simulink model "Fb_lin_control_hovering"  (R2021b)
settings: Solver=ode4  StartTime=0.0  StopTime=10.0  FixedStep=1e-4  RelTol=1e-3
settings Model: Creator=pierg  LastModifiedBy=pierg
settings ModelReferenceCC: ModelReferenceMinAlgLoopOccurrences=on

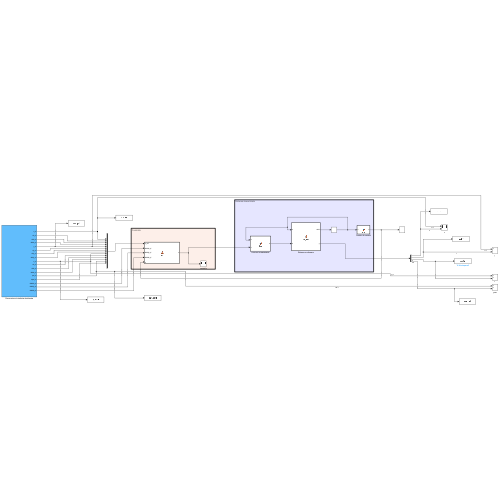
[thumbnail: Simulink's stored preview of the top-level diagram]
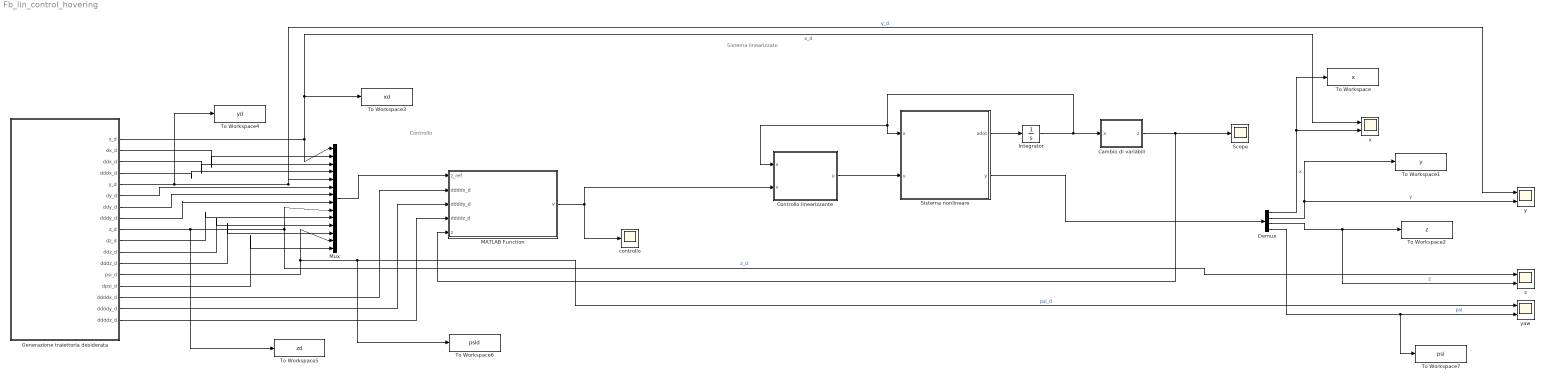
== system Fb_lin_control_hovering ==
  note: Controllo
  note: Sistema linearizzato
  Cambio di variabili : MATLAB Function  TreatAsAtomicUnit=on
  Controllo linearizzante : MATLAB Function  TreatAsAtomicUnit=on
  Demux : Demux
  Generazione traiettoria desiderata : Subsystem
  Integrator : Integrator  InitialCondition=[10 5 5 0 0 0 0 0 pi/4 0 0 0 9.81*2 0]'
  MATLAB Function : MATLAB Function  TreatAsAtomicUnit=on
  Mux : Mux  Inputs=14
  Scope : Scope
  Sistema nonlineare : MATLAB Function  TreatAsAtomicUnit=on
  To Workspace : ToWorkspace  VariableName=x  SaveFormat=Structure  SampleTime=-1
  To Workspace1 : ToWorkspace  VariableName=y  SaveFormat=Structure  SampleTime=-1
  To Workspace2 : ToWorkspace  VariableName=z  SaveFormat=Structure  SampleTime=-1
  To Workspace3 : ToWorkspace  VariableName=xd  SaveFormat=Structure  SampleTime=-1
  To Workspace4 : ToWorkspace  VariableName=yd  SaveFormat=Structure  SampleTime=-1
  To Workspace5 : ToWorkspace  VariableName=zd  SaveFormat=Structure  SampleTime=-1
  To Workspace6 : ToWorkspace  VariableName=psid  SaveFormat=Structure  SampleTime=-1
  To Workspace7 : ToWorkspace  VariableName=psi  SaveFormat=Structure  SampleTime=-1
  controllo : Scope
  x : Scope  NumInputPorts=2
  y : Scope  NumInputPorts=2
  yaw : Scope  NumInputPorts=2
  z : Scope  NumInputPorts=2
  wires:
  Sistema nonlineare/1(xdot) -> Integrator/1
  Integrator/1 -> Cambio di variabili/1(x), Controllo linearizzante/1(x), Sistema nonlineare/1(x)
  Controllo linearizzante/1(u) -> Sistema nonlineare/2(u)
  Sistema nonlineare/2(y) -> Demux/1
  Demux/1 -> To Workspace/1, x/2  "x"
  Demux/2 -> To Workspace1/1, y/2  "y"
  Demux/3 -> To Workspace2/1, z/2  "z"
  Cambio di variabili/1(z) -> MATLAB Function/5(z), Scope/1
  MATLAB Function/1(v) -> controllo/1, Controllo linearizzante/2(v)
  Generazione traiettoria desiderata/9(z_d) -> To Workspace5/1, Mux/9, z/1  "z_d"
  Generazione traiettoria desiderata/8(dddy_d) -> Mux/8
  Generazione traiettoria desiderata/10(dz_d) -> Mux/10
  Generazione traiettoria desiderata/7(ddy_d) -> Mux/7
  Generazione traiettoria desiderata/11(ddz_d) -> Mux/11
  Generazione traiettoria desiderata/6(dy_d) -> Mux/6
  Generazione traiettoria desiderata/12(dddz_d) -> Mux/12
  Generazione traiettoria desiderata/5(y_d) -> To Workspace4/1, y/1, Mux/5  "y_d"
  Generazione traiettoria desiderata/13(psi_d) -> To Workspace6/1, yaw/1, Mux/13  "psi_d"
  Generazione traiettoria desiderata/4(dddx_d) -> Mux/4
  Generazione traiettoria desiderata/14(dpsi_d) -> Mux/14
  Generazione traiettoria desiderata/3(ddx_d) -> Mux/3
  Generazione traiettoria desiderata/2(dx_d) -> Mux/2
  Generazione traiettoria desiderata/1(x_d) -> To Workspace3/1, x/1, Mux/1  "x_d"
  Mux/1 -> MATLAB Function/1(z_ref)
  Generazione traiettoria desiderata/15(ddddx_d) -> MATLAB Function/2(ddddx_d)
  Generazione traiettoria desiderata/16(ddddy_d) -> MATLAB Function/3(ddddy_d)
  Generazione traiettoria desiderata/17(ddddz_d) -> MATLAB Function/4(ddddz_d)
  Demux/4 -> To Workspace7/1, yaw/2  "psi"

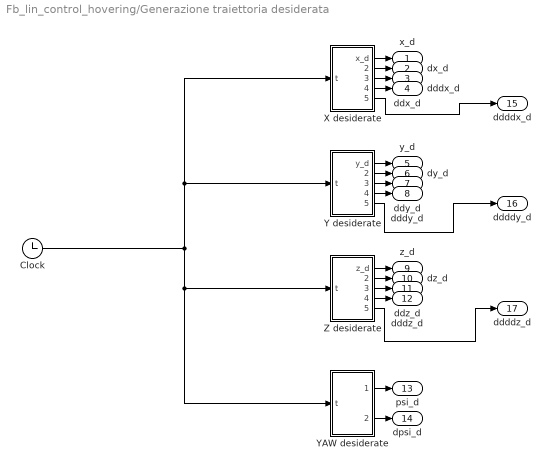
== system Fb_lin_control_hovering/Generazione traiettoria desiderata ==
  Clock : Clock
  X desiderate : Subsystem
  Y desiderate : Subsystem
  YAW desiderate : Subsystem
  Z desiderate : Subsystem
  x_d : Outport
  dx_d : Outport  Port=2
  ddx_d : Outport  Port=3
  dddx_d : Outport  Port=4
  y_d : Outport  Port=5
  dy_d : Outport  Port=6
  ddy_d : Outport  Port=7
  dddy_d : Outport  Port=8
  z_d : Outport  Port=9
  dz_d : Outport  Port=10
  ddz_d : Outport  Port=11
  dddz_d : Outport  Port=12
  psi_d : Outport  Port=13
  dpsi_d : Outport  Port=14
  ddddx_d : Outport  Port=15
  ddddy_d : Outport  Port=16
  ddddz_d : Outport  Port=17
  wires:
  Y desiderate/1(y_d) -> y_d/1
  Y desiderate/2(dy_d) -> dy_d/1
  X desiderate/5(ddddx_d) -> ddddx_d/1
  X desiderate/3(ddx_d) -> ddx_d/1
  YAW desiderate/2(dpsi_d) -> dpsi_d/1
  Z desiderate/1(z_d) -> z_d/1
  Z desiderate/4(dddz_d) -> dddz_d/1
  X desiderate/2(dx_d) -> dx_d/1
  Y desiderate/4(dddy_d) -> dddy_d/1
  X desiderate/4(dddx_d) -> dddx_d/1
  Y desiderate/3(ddy_d) -> ddy_d/1
  X desiderate/1(x_d) -> x_d/1
  Z desiderate/5(ddddz_d) -> ddddz_d/1
  Z desiderate/2(dz_d) -> dz_d/1
  YAW desiderate/1(psi_d) -> psi_d/1
  Z desiderate/3(ddz_d) -> ddz_d/1
  Y desiderate/5(ddddy_d) -> ddddy_d/1
  Clock/1 -> YAW desiderate/1(t), Z desiderate/1(t), X desiderate/1(t), Y desiderate/1(t)

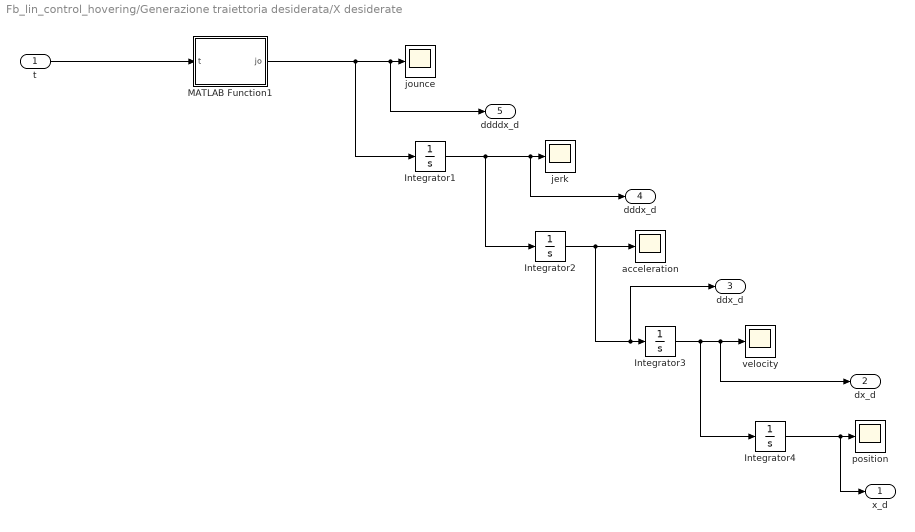
== system Fb_lin_control_hovering/Generazione traiettoria desiderata/X desiderate ==
  t : Inport
  Integrator1 : Integrator
  Integrator2 : Integrator
  Integrator3 : Integrator
  Integrator4 : Integrator  InitialCondition=10
  MATLAB Function1 : MATLAB Function  TreatAsAtomicUnit=on
  acceleration : Scope
  jerk : Scope
  jounce : Scope
  position : Scope
  velocity : Scope
  x_d : Outport
  dx_d : Outport  Port=2
  ddx_d : Outport  Port=3
  dddx_d : Outport  Port=4
  ddddx_d : Outport  Port=5
  wires:
  MATLAB Function1/1(jo) -> Integrator1/1, ddddx_d/1, jounce/1
  Integrator4/1 -> x_d/1, position/1
  Integrator3/1 -> Integrator4/1, dx_d/1, velocity/1
  Integrator2/1 -> ddx_d/1, Integrator3/1, acceleration/1
  Integrator1/1 -> Integrator2/1, dddx_d/1, jerk/1
  t/1 -> MATLAB Function1/1(t)

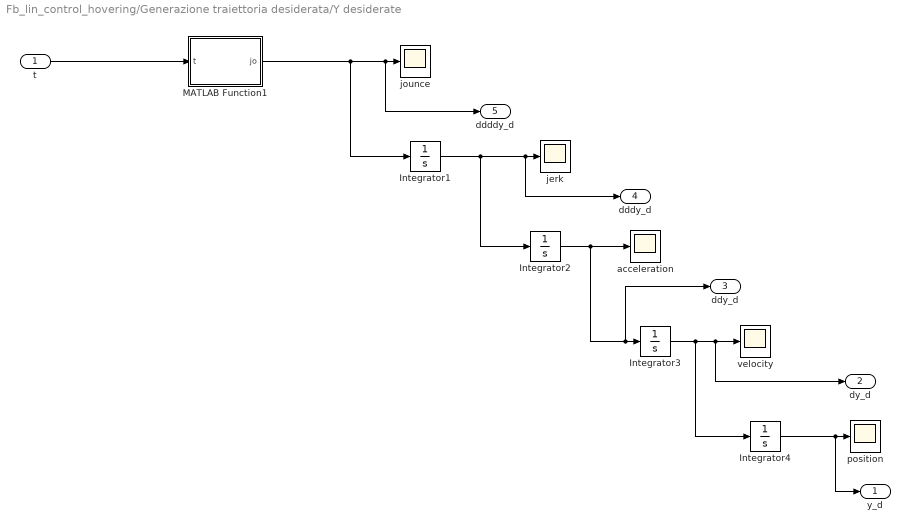
== system Fb_lin_control_hovering/Generazione traiettoria desiderata/Y desiderate ==
  t : Inport
  Integrator1 : Integrator
  Integrator2 : Integrator
  Integrator3 : Integrator
  Integrator4 : Integrator  InitialCondition=5
  MATLAB Function1 : MATLAB Function  TreatAsAtomicUnit=on
  acceleration : Scope
  jerk : Scope
  jounce : Scope
  position : Scope
  velocity : Scope
  y_d : Outport
  dy_d : Outport  Port=2
  ddy_d : Outport  Port=3
  dddy_d : Outport  Port=4
  ddddy_d : Outport  Port=5
  wires:
  t/1 -> MATLAB Function1/1(t)
  Integrator1/1 -> jerk/1, dddy_d/1, Integrator2/1
  Integrator2/1 -> acceleration/1, Integrator3/1, ddy_d/1
  Integrator3/1 -> velocity/1, dy_d/1, Integrator4/1
  Integrator4/1 -> position/1, y_d/1
  MATLAB Function1/1(jo) -> jounce/1, ddddy_d/1, Integrator1/1

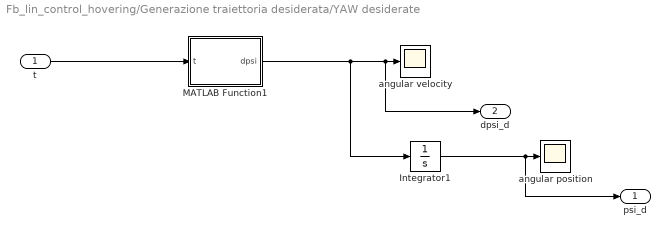
== system Fb_lin_control_hovering/Generazione traiettoria desiderata/YAW desiderate ==
  t : Inport
  Integrator1 : Integrator
  MATLAB Function1 : MATLAB Function  TreatAsAtomicUnit=on
  angular position : Scope
  angular velocity : Scope
  psi_d : Outport
  dpsi_d : Outport  Port=2
  wires:
  t/1 -> MATLAB Function1/1(t)
  Integrator1/1 -> angular position/1, psi_d/1
  MATLAB Function1/1(dpsi) -> angular velocity/1, dpsi_d/1, Integrator1/1

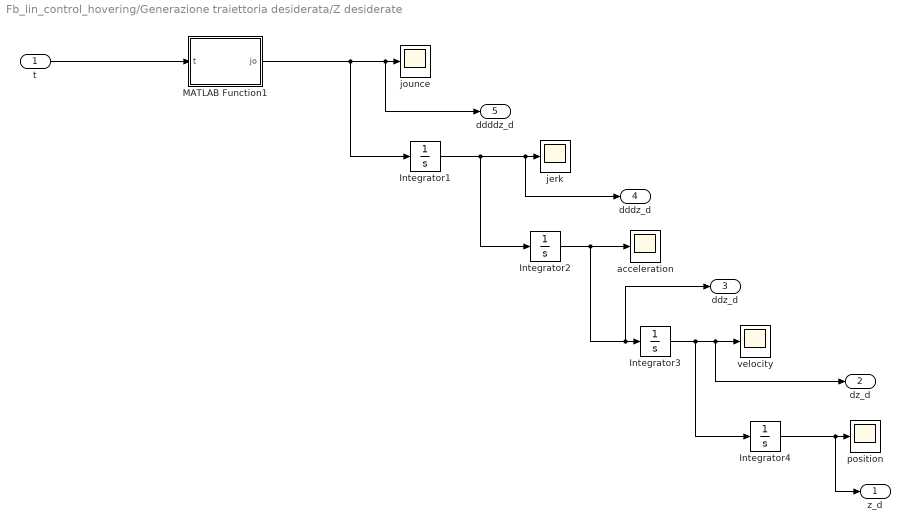
== system Fb_lin_control_hovering/Generazione traiettoria desiderata/Z desiderate ==
  t : Inport
  Integrator1 : Integrator
  Integrator2 : Integrator
  Integrator3 : Integrator
  Integrator4 : Integrator  InitialCondition=5
  MATLAB Function1 : MATLAB Function  TreatAsAtomicUnit=on
  acceleration : Scope
  jerk : Scope
  jounce : Scope
  position : Scope
  velocity : Scope
  z_d : Outport
  dz_d : Outport  Port=2
  ddz_d : Outport  Port=3
  dddz_d : Outport  Port=4
  ddddz_d : Outport  Port=5
  wires:
  MATLAB Function1/1(jo) -> Integrator1/1, ddddz_d/1, jounce/1
  Integrator4/1 -> z_d/1, position/1
  Integrator3/1 -> Integrator4/1, dz_d/1, velocity/1
  Integrator2/1 -> ddz_d/1, Integrator3/1, acceleration/1
  Integrator1/1 -> Integrator2/1, dddz_d/1, jerk/1
  t/1 -> MATLAB Function1/1(t)

== matlab function Fb_lin_control_hovering/Sistema nonlineare ==
  data: x input; u input; xdot output; y output
function [xdot, y] = nl_sys(x, u)
% Variabili di stato
x1 = x(1);
x2 = x(2);
x3 = x(3);
x4 = x(4);
x5 = x(5);
x6 = x(6);
x7 = x(7);
x8 = x(8);
x9 = x(9);
x10 = x(10);
x11 = x(11);
x12 = x(12);
u1 = x(13);
du1 = x(14);
% Ingressi di controllo
s1 = u(1);
u2 = u(2);
u3 = u(3);
u4 = u(4);
% Parametri
m = 2; % kg
g = 9.81; % m/s^2
Ix = 1.25; % kg*m^2
Iy = 1.25; % kg*m^2
Iz = 2.5; % kg*m^2
dwx = 0; %m/s^2
dwy = 0; %m/s^2
dwz = 0; %m/s^2

% Il sistema complessivo diventa
f_aa = [x4 x5 x6 -sin(x8)*u1/m sin(x7)*cos(x8)*u1/m -g+cos(x7)*cos(x8)*u1/m x10*cos(x9)-x11*sin(x9) x10*sin(x9)+x11*cos(x9) ...
    x12 0 0 0 du1 0]';
g1_aa = [0 0 0 0 0 0 0 0 0 0 0 0 0 1]';
g2_aa = [0 0 0 0 0 0 0 0 0 1/Ix 0 0 0 0]';
g3_aa = [0 0 0 0 0 0 0 0 0 0 1/Iy 0 0 0]';
g4_aa = [0 0 0 0 0 0 0 0 0 0 0 1/Iz 0 0]';

xdot = f_aa + g1_aa*s1 + g2_aa*u2 + g3_aa*u3 + g4_aa*u4;
y = [x1;x2;x3;x9];

== matlab function Fb_lin_control_hovering/Controllo linearizzante ==
  data: x input; u output; v input
function u = fcn(x, v)
% Variabili di stato
x1 = x(1);
x2 = x(2);
x3 = x(3);
x4 = x(4);
x5 = x(5);
x6 = x(6);
x7 = x(7);
x8 = x(8);
x9 = x(9);
x10 = x(10);
x11 = x(11);
x12 = x(12);
u1 = x(13);
du1 = x(14);
% Parametri
m = 2; % kg
g = 9.81; % m/s^2
Ix = 1.25; % kg*m^2
Iy = 1.25; % kg*m^2
Iz = 2.5; % kg*m^2
dwx = 0; %m/s^2
dwy = 0; %m/s^2
dwz = 0; %m/s^2

E = E_fun(Ix,Iy,Iz,m,u1,x7,x8,x9);
Gamma = Gamma_fun(du1,m,u1,x7,x8,x9,x10,x11,x12);

% Controllo necessario alla linearizzazione del modello a valle
u = -inv(E)*Gamma + inv(E)*v;

== matlab function Fb_lin_control_hovering/Cambio di variabili ==
  data: x input; z output
function z = fcn(x)
% Variabili di stato
x1 = x(1);
x2 = x(2);
x3 = x(3);
x4 = x(4);
x5 = x(5);
x6 = x(6);
x7 = x(7);
x8 = x(8);
x9 = x(9);
x10 = x(10);
x11 = x(11);
x12 = x(12);
u1 = x(13);
du1 = x(14);
% Parametri
m = 2; % kg
g = 9.81; % m/s^2
Ix = 1.25; % kg*m^2
Iy = 1.25; % kg*m^2
Iz = 2.5; % kg*m^2
dwx = 0; %m/s^2
dwy = 0; %m/s^2
dwz = 0; %m/s^2

z1 = x1; 
z2 = x4; 
z3 = -sin(x8)*u1/m; 
z4 = - (du1*sin(x8))/m - (u1*cos(x8)*(x11*cos(x9) + x10*sin(x9)))/m;  
z5 = x2; 
z6 = x5; 
z7 = sin(x7)*cos(x8)*u1/m; 
z8 = (du1*cos(x8)*sin(x7))/m + (u1*cos(x7)*cos(x8)*(x10*cos(x9) - x11*sin(x9)))/m - (u1*sin(x7)*sin(x8)*(x11*cos(x9) + x10*sin(x9)))/m;
z9 = x3; 
z10 = x6; 
z11 = cos(x7)*cos(x8)*u1/m - g; 
z12 = (du1*cos(x7)*cos(x8))/m - (u1*cos(x7)*sin(x8)*(x11*cos(x9) + x10*sin(x9)))/m - (u1*cos(x8)*sin(x7)*(x10*cos(x9) - x11*sin(x9)))/m;
z13 = x9; 
z14 = x12;

% Nuovo vettore di stato
z = [z1 z2 z3 z4 z5 z6 z7 z8 z9 z10 z11 z12 z13 z14]';

== matlab function Fb_lin_control_hovering/Generazione traiettoria desiderata/X desiderate/MATLAB Function1 ==
  data: t input; jo output
function jo = jounce(t)
% % Parametri
% a = 1;
% b = 1;
% c = 1;
% 
% % Accelerating part
% if t < b
%     j = a * sin(pi*t/b);
% elseif t >= b && t <= 3*b
%     j = -a * sin(pi*t/(2*b)-pi/2);
% elseif t > 3*b && t <= 4*b
%     j = a * sin(pi*t/b-3*pi);
% elseif t > 4*b && t <= 4*b+c
%     j = 0;
% % Decelerating part
% elseif t > 4*b+c && t <= 5*b+c
%     j = a * sin(pi*t/b);
% elseif t > 5*b+c && t <= 7*b+c
%     j = a * sin(0.5*pi*t/(b)+pi);
% elseif t > 7*b+c && t <= 8*b+c
%     j = a * sin(pi*t/b-3*pi);
% else
%     j = 0;
% end

jo = 0;

== matlab function Fb_lin_control_hovering/MATLAB Function ==
  data: z_ref input; ddddx_d input; ddddy_d input; ddddz_d input; z input; v output
function v = fcn(z_ref, ddddx_d, ddddy_d, ddddz_d, z)


% Definisco i riferimenti per l'uscita 1 (x)
e1 = z_ref(1:4) - z(1:4);
K1 = [18 30 20 4];
v1 = ddddx_d + K1*e1;
% Definisco i riferimenti per l'uscita 2 (y)
e2 = z_ref(5:8) - z(5:8);
K2 = [18 30 20 4];
v2 = ddddy_d + K2*e2;
% Definisco i riferimenti per l'uscita 3 (z)
e3 = z_ref(9:12) - z(9:12);
K3 = [15 30 20 4];
v3 = ddddz_d + K3*e3;
% Definisco i riferimenti per l'uscita 4 (yaw)
e4 = z_ref(13:14) - z(13:14);
K4 = [45 36];
v4 = K4*e4;

% Vettore dei riferimenti
v = [v1; v2; v3; v4];

== matlab function Fb_lin_control_hovering/Generazione traiettoria desiderata/Y desiderate/MATLAB Function1 ==
  data: t input; jo output
function jo = jounce(t)
% % Parametri
% a = 1/10;
% b = 1;
% c = 1;
% 
% % Accelerating part
% if t < b
%     j = a * sin(pi*t/b);
% elseif t >= b && t <= 3*b
%     j = -a * sin(pi*t/(2*b)-pi/2);
% elseif t > 3*b && t <= 4*b
%     j = a * sin(pi*t/b-3*pi);
% elseif t > 4*b && t <= 4*b+c
%     j = 0;
% % Decelerating part
% elseif t > 4*b+c && t <= 5*b+c
%     j = a * sin(pi*t/b);
% elseif t > 5*b+c && t <= 7*b+c
%     j = a * sin(0.5*pi*t/(b)+pi);
% elseif t > 7*b+c && t <= 8*b+c
%     j = a * sin(pi*t/b-3*pi);
% else
%     j = 0;
% end

jo = 0;

== matlab function Fb_lin_control_hovering/Generazione traiettoria desiderata/Z desiderate/MATLAB Function1 ==
  data: t input; jo output
function jo = jounce(t)
% Parametri
a = 1;
b = 1;
c = 1;

% Accelerating part
if t < b
    j = a * sin(pi*t/b);
elseif t >= b && t <= 3*b
    j = -a * sin(pi*t/(2*b)-pi/2);
elseif t > 3*b && t <= 4*b
    j = a * sin(pi*t/b-3*pi);
elseif t > 4*b && t <= 4*b+c
    j = 0;
% Decelerating part
elseif t > 4*b+c && t <= 5*b+c
    j = a * sin(pi*t/b);
elseif t > 5*b+c && t <= 7*b+c
    j = a * sin(0.5*pi*t/(b)+pi);
elseif t > 7*b+c && t <= 8*b+c
    j = a * sin(pi*t/b-3*pi);
else
    j = 0;
end

jo = j;

== matlab function Fb_lin_control_hovering/Generazione traiettoria desiderata/YAW desiderate/MATLAB Function1 ==
  data: t input; dpsi output
function dpsi = ang_vel(t)
% % Parametri
% a = 1/3;
% b = 2;
% c =2;
% 
% % Accelerating part
% if t < b
%     j = a * sin(pi*t/b);
% elseif t >= b && t <= 3*b
%     j = -a * sin(pi*t/(2*b)-pi/2);
% elseif t > 3*b && t <= 4*b
%     j = a * sin(pi*t/b-3*pi);
% elseif t > 4*b && t <= 4*b+c
%     j = 0;
% % Decelerating part
% elseif t > 4*b+c && t <= 5*b+c
%     j = a * sin(pi*t/b);
% elseif t > 5*b+c && t <= 7*b+c
%     j = a * sin(0.5*pi*t/(b)+pi);
% elseif t > 7*b+c && t <= 8*b+c
%     j = a * sin(pi*t/b-3*pi);
% else
%     j = 0;
% end

dpsi = 0*t;
